simulink model "filecuaho"  (R2016b)
settings: Solver=VariableStepAuto  StartTime=0.0  StopTime=10.0  RelTol=1e-3
undefined symbols (not defined in the file): KACC_ACCT_CLR_NIDL_INIT, KACC_ACCUT_STATE_A, KACC_ACCUT_STATE_B, KACC_ACCUT_SW, KACC_ACTQSW, KACC_CLD, KACC_CLD_REQ_HYS, KACC_CLD_REQ_SW, KACC_COLPD, KACC_COMP_INRT, KACC_COMPTYPE_FIXED, KACC_COMPTYPE_VAR, KACC_CTTM_ACE, KACC_CTTM_ACON, KACC_CTTM_CRK, KACC_CTTM_FAN, KACC_CTTM_GRD, KACC_CTTM_IRS, KACC_CTTM_NAC, KACC_DIFFEVATEMPMAX, KACC_DIFFEVATEMPMIN, KACC_EVAT_ELSE, KACC_EVAT_ELSE_SW, KACC_EVATMPCUT_SW, KACC_EVATUPL_ELSE, KACC_EVATUPL_ELSE_SW, KACC_FANREQ_SW, KACC_FORCEDACON, KACC_HCAPS, KACC_HCAPS_HYS, KACC_HCCTTM, KACC_HCGRA, KACC_HCGRA_HYS, KACC_HCRGR, KACC_HCVS1, KACC_HCVS1_HYS, KACC_HCVS2, KACC_HCVS2_HYS, KACC_HEATUP_CE, KACC_HEATUP_CE_HYS, KACC_HEATUP_DRV2IDL, KACC_HEATUP_IDL2DRV, KACC_HEATUP_NE, KACC_HEATUP_NE_HYS, KACC_HIPS_ACOF, KACC_HIPS_ACON, KACC_LOPS_ACOF, KACC_LOPS_ACON, KACC_LYR3TR_ACHLD, KACC_NEW_RPM, KACC_OFDL_SW, KACC_OFDL_VCV, KACC_ONDL_SW, KACC_RECCP, KACC_RECCP_HYS, KACC_RECDLY, KACC_RECVS, KACC_S1_THWMAX, KACC_S1TM_THWULMT, KACC_SHLT_2CYL ... (+137)
libraries: lib2011b x727, SUBSYSTEM_LIB_CNV x30, SUBSYSTEM_LIB_ESC x2, SUBSYSTEM_LIB_AUX x1
(part 2 of 5)

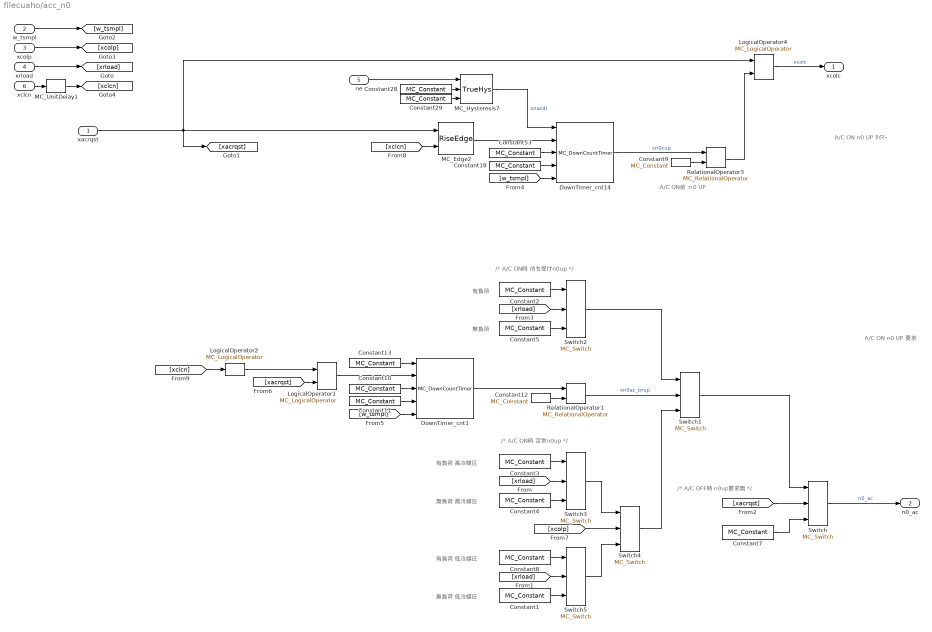
== system filecuaho/acc_n0 ==
  note: A/C ON前 ｎ0 UP
  note: A/C ON
      | n0 UP ﾀｲﾏｰ
  note: A/C ON
      | n0 UP 要求
  note: /* A/C ON時 待ち受けn0up */
  note: /* A/C ON時 定常n0up */
  note: /* A/C OFF時 n0up要求無 */
  note: 有負荷 高冷媒圧
  note: 無負荷 高冷媒圧
  note: 有負荷 低冷媒圧
  note: 無負荷 低冷媒圧
  note: 有負荷
  note: 無負荷
  xacrqst : Inport
  w_tsmpl : Inport  Port=2
  xcolp : Inport  Port=3
  xrload : Inport  Port=4
  ne : Inport  Port=5
  xclcn : Inport  Port=6
  Constant1 : lib2011b/Simulink Original/Sources/MC_Constant  Value=KINLCN  datatype=Inherit: Inherit from 'Constant value'  SampleTime=inf  FramePeriod=inf  OutMin=[]  OutMax=[]  OutDataTypeStr=Inherit: Inherit from 'Constant value'
  Constant10 : lib2011b/Simulink Original/Sources/MC_Constant  Value=true  datatype=Inherit: Inherit from 'Constant value'  SampleTime=inf  FramePeriod=inf  OutMin=[]  OutMax=[]  OutDataTypeStr=Inherit: Inherit from 'Constant value'
  Constant11 : lib2011b/Simulink Original/Sources/MC_Constant  Value=KLN0BRUP  datatype=Inherit: Inherit from 'Constant value'  SampleTime=inf  FramePeriod=inf  OutMin=[]  OutMax=[]  OutDataTypeStr=Inherit: Inherit from 'Constant value'
  Constant12 : lib2011b/Simulink Original/Sources/MC_Constant  Value=0  datatype=single  SampleTime=inf  FramePeriod=inf  OutMin=[]  OutMax=[]  OutDataTypeStr=single
  Constant13 : lib2011b/Simulink Original/Sources/MC_Constant  Value=false  datatype=Inherit: Inherit from 'Constant value'  SampleTime=inf  FramePeriod=inf  OutMin=[]  OutMax=[]  OutDataTypeStr=Inherit: Inherit from 'Constant value'
  Constant18 : lib2011b/Simulink Original/Sources/MC_Constant  Value=KLN0CUP  datatype=Inherit: Inherit from 'Constant value'  SampleTime=inf  FramePeriod=inf  OutMin=[]  OutMax=[]  OutDataTypeStr=Inherit: Inherit from 'Constant value'
  Constant2 : lib2011b/Simulink Original/Sources/MC_Constant  Value=KINLC1  datatype=Inherit: Inherit from 'Constant value'  SampleTime=inf  FramePeriod=inf  OutMin=[]  OutMax=[]  OutDataTypeStr=Inherit: Inherit from 'Constant value'
  Constant28 : lib2011b/Simulink Original/Sources/MC_Constant  Value=KSNACDL  datatype=Inherit: Inherit from 'Constant value'  SampleTime=inf  FramePeriod=inf  OutMin=[]  OutMax=[]  OutDataTypeStr=Inherit: Inherit from 'Constant value'
  Constant29 : lib2011b/Simulink Original/Sources/MC_Constant  Value=KSNACDL_HYS  datatype=Inherit: Inherit from 'Constant value'  SampleTime=inf  FramePeriod=inf  OutMin=[]  OutMax=[]  OutDataTypeStr=Inherit: Inherit from 'Constant value'
  Constant3 : lib2011b/Simulink Original/Sources/MC_Constant  Value=KINLCH  datatype=Inherit: Inherit from 'Constant value'  SampleTime=inf  FramePeriod=inf  OutMin=[]  OutMax=[]  OutDataTypeStr=Inherit: Inherit from 'Constant value'
  Constant4 : lib2011b/Simulink Original/Sources/MC_Constant  Value=KINLCHN  datatype=Inherit: Inherit from 'Constant value'  SampleTime=inf  FramePeriod=inf  OutMin=[]  OutMax=[]  OutDataTypeStr=Inherit: Inherit from 'Constant value'
  Constant5 : lib2011b/Simulink Original/Sources/MC_Constant  Value=KINLC1N  datatype=Inherit: Inherit from 'Constant value'  SampleTime=inf  FramePeriod=inf  OutMin=[]  OutMax=[]  OutDataTypeStr=Inherit: Inherit from 'Constant value'
  Constant53 : lib2011b/Simulink Original/Sources/MC_Constant  Value=true  datatype=Inherit: Inherit from 'Constant value'  SampleTime=inf  FramePeriod=inf  OutMin=[]  OutMax=[]  OutDataTypeStr=Inherit: Inherit from 'Constant value'
  Constant7 : lib2011b/Simulink Original/Sources/MC_Constant  Value=0  datatype=single  SampleTime=inf  FramePeriod=inf  OutMin=[]  OutMax=[]  OutDataTypeStr=single
  Constant8 : lib2011b/Simulink Original/Sources/MC_Constant  Value=KINLC  datatype=Inherit: Inherit from 'Constant value'  SampleTime=inf  FramePeriod=inf  OutMin=[]  OutMax=[]  OutDataTypeStr=Inherit: Inherit from 'Constant value'
  Constant9 : lib2011b/Simulink Original/Sources/MC_Constant  Value=0  datatype=single  SampleTime=inf  FramePeriod=inf  OutMin=[]  OutMax=[]  OutDataTypeStr=single
  DownTimer_cnt1 : lib2011b/Mazda Library/Timer/MC_DownCountTimer
      settings: AttributesFormatString=DownCountTimer
  DownTimer_cnt14 : lib2011b/Mazda Library/Timer/MC_DownCountTimer
      settings: AttributesFormatString=DownCountTimer
  LogicalOperator1 : lib2011b/Simulink Original/Logic and Bit Operations/MC_LogicalOperator  SelectedOperator=AND  Inputs=2  SampleTime=-1  AllPortsSameDT=off  OutDataTypeStr=boolean
  LogicalOperator2 : lib2011b/Simulink Original/Logic and Bit Operations/MC_LogicalOperator  SelectedOperator=NOT  Inputs=2  SampleTime=-1  AllPortsSameDT=off  OutDataTypeStr=boolean
  LogicalOperator4 : lib2011b/Simulink Original/Logic and Bit Operations/MC_LogicalOperator  SelectedOperator=AND  Inputs=2  SampleTime=-1  AllPortsSameDT=off  OutDataTypeStr=boolean
  MC_Edge2 : SUBSYSTEM_LIB_CNV/RiseEdge
      settings: AttributesFormatString=RISE
  MC_Hysteresis7 : SUBSYSTEM_LIB_CNV/TrueHys
      settings: AttributesFormatString=True
  MC_UnitDelay1 : lib2011b/Simulink Original/Discrete/MC_UnitDelay  InitialCondition=0  InputProcessing=Inherited  SampleTime=-1  StateName=delay_yclcn_b20m9489
      settings: StateMustResolveToSignalObject=off  StateStorageClass=ExportedGlobal
  RelationalOperator1 : lib2011b/Simulink Original/Logic and Bit Operations/MC_RelationalOperator  Operator=>  SampleTime=-1  InputSameDT=on  OutDataTypeStr=boolean
  RelationalOperator3 : lib2011b/Simulink Original/Logic and Bit Operations/MC_RelationalOperator  Operator=<=  SampleTime=-1  InputSameDT=on  OutDataTypeStr=boolean
  Switch{,1..5} (6 alike) : lib2011b/Simulink Original/Signal Routing/MC_Switch  Criteria=u2 ~= 0  Threshold=0  SampleTime=-1  InputSameDT=on  OutMin=[]  OutMax=[]  AllowDiffInputSizes=off
  xcolc : Outport
  n0_ac : Outport  Port=2
  wires:
  RelationalOperator3/1 -> LogicalOperator4/2
  Constant9/1 -> RelationalOperator3/2
  ne/1 -> MC_Hysteresis7/1
  Constant28/1 -> MC_Hysteresis7/2
  Constant29/1 -> MC_Hysteresis7/3
  xacrqst/1 -> MC_Edge2/1, LogicalOperator4/1, [xacrqst]
  MC_Edge2/1 -> DownTimer_cnt14/2
  MC_Hysteresis7/1 -> DownTimer_cnt14/1  "xnacdl"
  Constant18/1 -> DownTimer_cnt14/4
  Constant53/1 -> DownTimer_cnt14/3
  DownTimer_cnt14/1 -> RelationalOperator3/1  "cn0cup"
  Switch/1 -> n0_ac/1  "n0_ac"
  Switch5/1 -> Switch4/3
  Switch3/1 -> Switch4/1
  Constant8/1 -> Switch5/1
  Constant1/1 -> Switch5/3
  Constant7/1 -> Switch/3
  Constant3/1 -> Switch3/1
  Constant4/1 -> Switch3/3
  xrload/1 -> [xrload]
  [xrload] -> Switch3/2
  [xrload] -> Switch5/2
  [xacrqst] -> Switch/2
  Switch4/1 -> Switch1/3
  Switch1/1 -> Switch/1
  Constant2/1 -> Switch2/1
  [xrload] -> Switch2/2
  Constant5/1 -> Switch2/3
  w_tsmpl/1 -> [w_tsmpl]
  [w_tsmpl] -> DownTimer_cnt14/5
  [w_tsmpl] -> DownTimer_cnt1/5
  Constant10/1 -> DownTimer_cnt1/3
  Constant11/1 -> DownTimer_cnt1/4
  Constant12/1 -> RelationalOperator1/2
  DownTimer_cnt1/1 -> RelationalOperator1/1
  Constant13/1 -> DownTimer_cnt1/1
  LogicalOperator1/1 -> DownTimer_cnt1/2
  LogicalOperator2/1 -> LogicalOperator1/1
  [xacrqst] -> LogicalOperator1/2
  RelationalOperator1/1 -> Switch1/2  "xn0ac_brup"
  xcolp/1 -> [xcolp]
  [xcolp] -> Switch4/2
  Switch2/1 -> Switch1/1
  xclcn/1 -> MC_UnitDelay1/1
  [xclcn] -> LogicalOperator2/1
  MC_UnitDelay1/1 -> [xclcn]
  [xclcn] -> MC_Edge2/2
  LogicalOperator4/1 -> xcolc/1  "xcolc"

== system filecuaho/acc_nidle_enable ==
  note: << 暖房性能要求 N-Idle禁止制御 >>
  note: ②暖房性能要求熱量(リニアインテーク補正後)=0
  note: インマニ温(tham)センサ回路故障時は
      | インマニ温度履歴が正しくないため許可判定をキャンセルする
  note: ③センサ故障時
  note: ①インマニ温熱履歴条件
  note: 水温(thw)
      | ↑
      | ｜／／／／／／／／／／／／／／／／｜
      | ｜(B)エンジンルームの放熱量によらず
      | ｜N-IDLE許可可能領域／／／／／／／
      | ｜／／／／／／／／／／／／／／／／｜
      | ｜――――――――――――――――＋― TWNIDL_HEAT(_HYS)
      | ｜××××××××××××××××｜ 　　　↑
      | ｜(C)アイドル時のエンジンルームへの放熱量が　　暖房性能要求熱量=0
      | ｜少ない場合N-IDLE許可可能領域××　　　　(リニアインテーク補正後)
      | ｜××××××××××××××××｜　　 　↓
      | ｜――――――――――――――――＋――――――
      | ｜　　　　　　　　　　　　　　　　　　　　　　　　｜
      | ｜(D)暖房性能よりN-IDLE禁止領域　　　　　→(A)暖房性能からの要求無
      | ｜　　　　　　　　　　　　　　　　　　　　　　　　｜
      | ＋―――――――――――――――――――→始動時水温(thws)
      | 　　　　　　　　　　　　　　　　KWNIDL_HEAT_STA
  note: ----------------(B)エンジンルームの放熱量によらずN-IDLE許可可能領域----------------
  note: ----------------(C)アイドル時のエンジンルームへの放熱量が少ない場合N-IDLE許可可能領域----------------
  note: ----------------(A)暖房性能からのN-IDLE禁止要求無----------------
  note: 10000
  note: 1
  note: ②暖房性能要求熱量(リニアインテーク補正後)<=所定値
  thw : Inport
  thws : Inport  Port=2
  thaa : Inport  Port=3
  des_heat_acc_gain_drv : Inport  Port=4
  xheat_cldvvt_req : Inport  Port=5
  tham : Inport  Port=6
  xthamcf : Inport  Port=7
  vspe : Inport  Port=8
  xbrst : Inport  Port=9
  w_tsmpl : Inport  Port=10
  FalseHys : SUBSYSTEM_LIB_CNV/FalseHys
      settings: AttributesFormatString=False
  MC_Add : lib2011b/Simulink Original/Math Operations/MC_Add  Inputs=+-  CollapseDim=1  SampleTime=-1  InputSameDT=on  OutMin=[]  OutMax=[]  OutDataTypeStr=single
  MC_Constant1 : lib2011b/Simulink Original/Sources/MC_Constant  Value=KWNIDL_HEAT_GAIN_SW  datatype=Inherit: Inherit from 'Constant value'  SampleTime=inf  FramePeriod=inf  OutMin=[]  OutMax=[]  OutDataTypeStr=Inherit: Inherit from 'Constant value'
  MC_Constant14 : lib2011b/Simulink Original/Sources/MC_Constant  Value=KWNIDL_HEAT_GAIN2  datatype=Inherit: Inherit from 'Constant value'  SampleTime=inf  FramePeriod=inf  OutMin=[]  OutMax=[]  OutDataTypeStr=Inherit: Inherit from 'Constant value'
  MC_Constant16 : lib2011b/Simulink Original/Sources/MC_Constant  Value=KWNIDL_HEAT_GAIN2_HYS  datatype=Inherit: Inherit from 'Constant value'  SampleTime=inf  FramePeriod=inf  OutMin=[]  OutMax=[]  OutDataTypeStr=Inherit: Inherit from 'Constant value'
  MC_Constant2 : lib2011b/Simulink Original/Sources/MC_Constant  Value=KWNIDL_HEAT_STA  datatype=Inherit: Inherit from 'Constant value'  SampleTime=inf  FramePeriod=inf  OutMin=[]  OutMax=[]  OutDataTypeStr=Inherit: Inherit from 'Constant value'
  MC_Constant3 : lib2011b/Simulink Original/Sources/MC_Constant  Value=KWNIDL_HEAT_GAIN  datatype=Inherit: Inherit from 'Constant value'  SampleTime=inf  FramePeriod=inf  OutMin=[]  OutMax=[]  OutDataTypeStr=Inherit: Inherit from 'Constant value'
  MC_Constant4 : lib2011b/Simulink Original/Sources/MC_Constant  Value=KWNIDL_HEAT_HYS  datatype=Inherit: Inherit from 'Constant value'  SampleTime=inf  FramePeriod=inf  OutMin=[]  OutMax=[]  OutDataTypeStr=Inherit: Inherit from 'Constant value'
  MC_Constant6 : lib2011b/Simulink Original/Sources/MC_Constant  Value=KWNIDL_LATCH_VSP  datatype=Inherit: Inherit from 'Constant value'  SampleTime=inf  FramePeriod=inf  OutMin=[]  OutMax=[]  OutDataTypeStr=Inherit: Inherit from 'Constant value'
  MC_Constant7 : lib2011b/Simulink Original/Sources/MC_Constant  Value=KWNIDL_THAM_FIL_TC  datatype=Inherit: Inherit from 'Constant value'  SampleTime=inf  FramePeriod=inf  OutMin=[]  OutMax=[]  OutDataTypeStr=Inherit: Inherit from 'Constant value'
  MC_DataTypeConversion1 : lib2011b/Simulink Original/Signal Attributes/MC_DataTypeConversion  OutMin=[]  OutMax=[]  OutDataTypeStr=boolean  Signaltype=boolean  ConvertRealWorld=Real World Value (RWV)  RndMeth=Zero  SaturateOnIntegerOverflow=on  SampleTime=-1
  MC_Hysteresis : SUBSYSTEM_LIB_CNV/TrueHys
      settings: AttributesFormatString=True
  MC_LogicalOperator1 : lib2011b/Simulink Original/Logic and Bit Operations/MC_LogicalOperator  SelectedOperator=AND  Inputs=3  SampleTime=-1  AllPortsSameDT=off  OutDataTypeStr=boolean
  MC_LogicalOperator2 : lib2011b/Simulink Original/Logic and Bit Operations/MC_LogicalOperator  SelectedOperator=NOT  Inputs=1  SampleTime=-1  AllPortsSameDT=off  OutDataTypeStr=boolean
  MC_LogicalOperator3 : lib2011b/Simulink Original/Logic and Bit Operations/MC_LogicalOperator  SelectedOperator=OR  Inputs=3  SampleTime=-1  AllPortsSameDT=off  OutDataTypeStr=boolean
  MC_LogicalOperator4 : lib2011b/Simulink Original/Logic and Bit Operations/MC_LogicalOperator  SelectedOperator=OR  Inputs=2  SampleTime=-1  AllPortsSameDT=off  OutDataTypeStr=boolean
  MC_LogicalOperator6 : lib2011b/Simulink Original/Logic and Bit Operations/MC_LogicalOperator  SelectedOperator=NOT  Inputs=1  SampleTime=-1  AllPortsSameDT=off  OutDataTypeStr=boolean
  MC_LowPassFilter : lib2011b/Mazda Library/Filter/MC_LowPassFilter
  MC_MinMax : lib2011b/Simulink Original/Math Operations/MC_MinMax  Function=min  Inputs=2  SampleTime=-1  InputSameDT=on  OutMin=[]  OutMax=[]
  MC_MinMax1 : lib2011b/Simulink Original/Math Operations/MC_MinMax  Function=min  Inputs=2  SampleTime=-1  InputSameDT=on  OutMin=[]  OutMax=[]
  MC_RelationalOperator : lib2011b/Simulink Original/Logic and Bit Operations/MC_RelationalOperator  Operator=>=  SampleTime=-1  InputSameDT=on  OutDataTypeStr=boolean
  MC_RelationalOperator1 : lib2011b/Simulink Original/Logic and Bit Operations/MC_RelationalOperator  Operator=<=  SampleTime=-1  InputSameDT=on  OutDataTypeStr=boolean
  MC_RelationalOperator2 : lib2011b/Simulink Original/Logic and Bit Operations/MC_RelationalOperator  Operator=>=  SampleTime=-1  InputSameDT=on  OutDataTypeStr=boolean
  MC_RelationalOperator4 : lib2011b/Simulink Original/Logic and Bit Operations/MC_RelationalOperator  Operator=>=  SampleTime=-1  InputSameDT=on  OutDataTypeStr=boolean
  MC_Switch1 : lib2011b/Simulink Original/Signal Routing/MC_Switch  Criteria=u2 ~= 0  Threshold=0  SampleTime=-1  InputSameDT=on  OutMin=[]  OutMax=[]  AllowDiffInputSizes=off
  MC_Switch2 : lib2011b/Simulink Original/Signal Routing/MC_Switch  Criteria=u2 ~= 0  Threshold=0  SampleTime=-1  InputSameDT=on  OutMin=[]  OutMax=[]  AllowDiffInputSizes=off
  MC_Table : lib2011b/Simulink Original/Lookup Tables/MC_Table_i  Label=TWNIDL_HEAT  InputValues=TWNIDL_HEAT_X  calsw_x=on  OutputValues=TWNIDL_HEAT_Y  LsbValue=LSB_TWNIDL_HEAT_Y  OffsetValue=OFFSET_TWNIDL_HEAT_Y
      settings: AttributesFormatString=%<Label>\nX-axis %<calsw_x>
  MC_Table1 : lib2011b/Simulink Original/Lookup Tables/MC_Table_i  Label=TWNIDL_DLT_THAM  InputValues=TWNIDL_DLT_THAM_X  calsw_x=on  OutputValues=TWNIDL_DLT_THAM_Y  LsbValue=LSB_TWNIDL_DLT_THAM_Y  OffsetValue=OFFSET_TWNIDL_DLT_THAM_Y
      settings: AttributesFormatString=%<Label>\nX-axis %<calsw_x>
  MC_UnitDelay : lib2011b/Simulink Original/Discrete/MC_UnitDelay  InitialCondition=0  InputProcessing=Inherited  SampleTime=-1  StateName=delay_yclcn_b20m9490
      settings: StateMustResolveToSignalObject=off  StateStorageClass=ExportedGlobal
  MC_UnitDelay1 : lib2011b/Simulink Original/Discrete/MC_UnitDelay  InitialCondition=0  InputProcessing=Inherited  SampleTime=-1  StateName=delay_yclcn_b20m9491
      settings: StateMustResolveToSignalObject=off  StateStorageClass=ExportedGlobal
  MC_UnitDelay3 : lib2011b/Simulink Original/Discrete/MC_UnitDelay  InitialCondition=0  InputProcessing=Inherited  SampleTime=-1  StateName=delay_yclcn_b20m9492
      settings: StateMustResolveToSignalObject=off  StateStorageClass=ExportedGlobal
  xnidle_ena_heat : Outport
  wires:
  thw/1 -> [thw]
  MC_Table/1 -> MC_Hysteresis/2
  MC_Constant4/1 -> MC_Hysteresis/3
  MC_Hysteresis/1 -> MC_LogicalOperator3/2
  thws/1 -> [thws]
  MC_Constant2/1 -> MC_RelationalOperator/2
  MC_RelationalOperator/1 -> MC_LogicalOperator3/1
  MC_MinMax/1 -> MC_Table/1, MC_UnitDelay/1
  thaa/1 -> MC_MinMax/1
  MC_UnitDelay/1 -> MC_MinMax/2
  MC_LogicalOperator3/1 -> xnidle_ena_heat/1  "xnidle_ena_heat"
  MC_UnitDelay1/1 -> MC_MinMax1/2
  MC_LowPassFilter/1 -> MC_MinMax1/1, MC_Add/1  "tham_fil_heat"
  MC_MinMax1/1 -> MC_UnitDelay1/1, MC_Add/2
  [thw] -> MC_Hysteresis/1
  [thws] -> MC_RelationalOperator/1
  MC_Add/1 -> MC_RelationalOperator2/1
  xthamcf/1 -> MC_LogicalOperator6/1
  MC_LogicalOperator6/1 -> MC_LogicalOperator1/3
  MC_Constant7/1 -> MC_LowPassFilter/2
  xbrst/1 -> MC_LowPassFilter/4
  w_tsmpl/1 -> MC_LowPassFilter/3
  tham/1 -> MC_LowPassFilter/1
  MC_Switch2/1 -> MC_UnitDelay3/1, MC_LogicalOperator3/3
  MC_UnitDelay3/1 -> MC_Switch2/3
  vspe/1 -> MC_RelationalOperator4/1
  MC_RelationalOperator4/1 -> MC_Switch2/2
  MC_Constant6/1 -> MC_RelationalOperator4/2
  xheat_cldvvt_req/1 -> MC_LogicalOperator2/1
  MC_Table1/1 -> MC_RelationalOperator2/2
  MC_RelationalOperator2/1 -> MC_LogicalOperator1/1
  MC_LogicalOperator1/1 -> MC_Switch2/1
  [thws] -> MC_Table1/1
  MC_Constant1/1 -> MC_DataTypeConversion1/1
  MC_DataTypeConversion1/1 -> MC_Switch1/2
  MC_Constant14/1 -> FalseHys/2
  MC_Constant16/1 -> FalseHys/3
  des_heat_acc_gain_drv/1 -> FalseHys/1, MC_RelationalOperator1/1
  MC_LogicalOperator4/1 -> MC_Switch1/1
  FalseHys/1 -> MC_LogicalOperator4/1
  MC_RelationalOperator1/1 -> MC_LogicalOperator4/2
  MC_Constant3/1 -> MC_RelationalOperator1/2
  MC_LogicalOperator2/1 -> MC_Switch1/3
  MC_Switch1/1 -> MC_LogicalOperator1/2

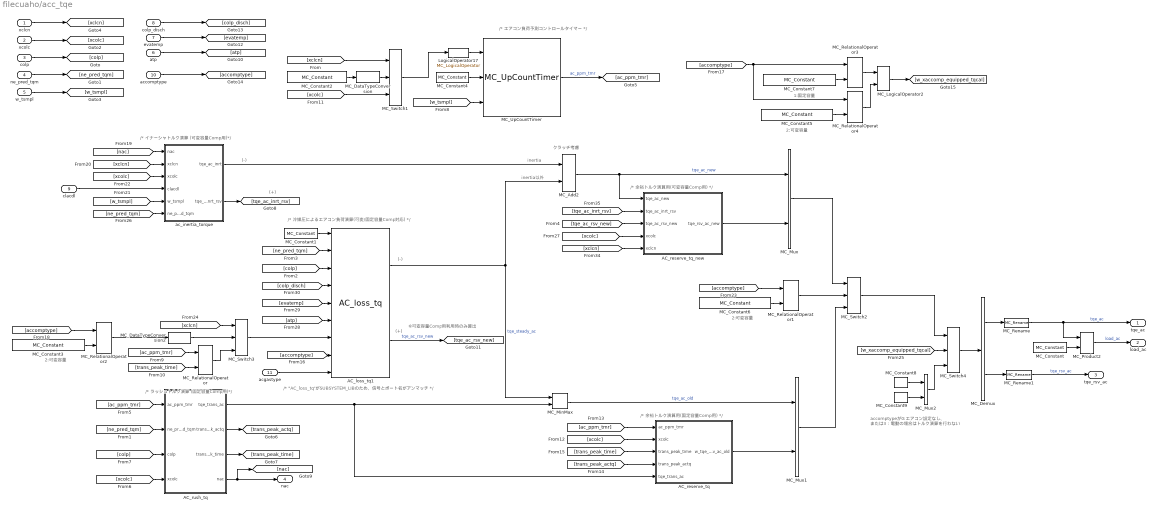
== system filecuaho/acc_tqe ==
  note: /* エアコン負荷予測コントロールタイマー */
  note: /* ラッシュトルク演算 (固定容量Comp用)*/
  note: /* 冷媒圧によるエアコン負荷演算(可変/固定容量Comp対応) */
  note: /* "AC_loss_tq"がSUBSYSTEM_LIBのため、信号とポート名がアンマッチ */
  note: /* 余裕トルク演算用(固定容量Comp用) */
  note: クラッチ考慮
  note: /* イナーシャトルク演算 (可変容量Comp用)*/
  note: inertia
  note: inertia以外
  note: (+)
  note: (-)
  note: (+)
  note: (-)
  note: /* 余裕トルク演算用(可変容量Comp用) */
  note: ※可変容量Comp用利用時のみ算出
  note: 2:可変容量
  note: 2:可変容量
  note: 2:可変容量
  note: 1:固定容量
  note: accomptypeが0:エアコン設定なし、
      | または3：電動の場合はトルク演算を行わない
  xclcn : Inport
  xcolc : Inport  Port=2
  colp : Inport  Port=3
  ne_pred_tqm : Inport  Port=4
  w_tsmpl : Inport  Port=5
  atp : Inport  Port=6
  evatemp : Inport  Port=7
  colp_disch : Inport  Port=8
  clacdl : Inport  Port=9
  accomptype : Inport  Port=10
  acgastype : Inport  Port=11
  AC_loss_tq1 : SUBSYSTEM_LIB_AUX/ACC/AC_loss_tq
  AC_reserve_tq : Subsystem
  AC_reserve_tq_new : Subsystem
  AC_rush_tq : Subsystem
  LogicalOperator17 : lib2011b/Simulink Original/Logic and Bit Operations/MC_LogicalOperator  SelectedOperator=NOT  Inputs=1  SampleTime=-1  AllPortsSameDT=off  OutDataTypeStr=boolean
  MC_Add2 : lib2011b/Simulink Original/Math Operations/MC_Add  Inputs=++  CollapseDim=1  SampleTime=-1  InputSameDT=on  OutMin=[]  OutMax=[]  OutDataTypeStr=single
  MC_Constant : lib2011b/Simulink Original/Sources/MC_Constant  Value=-1  datatype=single  SampleTime=inf  FramePeriod=inf  OutMin=[]  OutMax=[]  OutDataTypeStr=single
  MC_Constant1 : lib2011b/Simulink Original/Sources/MC_Constant  Value=1  datatype=single  SampleTime=inf  FramePeriod=inf  OutMin=[]  OutMax=[]  OutDataTypeStr=single
  MC_Constant2 : lib2011b/Simulink Original/Sources/MC_Constant  Value=KACC_ACTQSW  datatype=Inherit: Inherit from 'Constant value'  SampleTime=inf  FramePeriod=inf  OutMin=[]  OutMax=[]  OutDataTypeStr=Inherit: Inherit from 'Constant value'
  MC_Constant3 : lib2011b/Simulink Original/Sources/MC_Constant  Value=KACC_COMPTYPE_VAR  datatype=Inherit: Inherit from 'Constant value'  SampleTime=inf  FramePeriod=inf  OutMin=[]  OutMax=[]  OutDataTypeStr=Inherit: Inherit from 'Constant value'
  MC_Constant4 : lib2011b/Simulink Original/Sources/MC_Constant  Value=true  datatype=Inherit: Inherit from 'Constant value'  SampleTime=inf  FramePeriod=inf  OutMin=[]  OutMax=[]  OutDataTypeStr=Inherit: Inherit from 'Constant value'
  MC_Constant5 : lib2011b/Simulink Original/Sources/MC_Constant  Value=KACC_COMPTYPE_VAR  datatype=Inherit: Inherit from 'Constant value'  SampleTime=inf  FramePeriod=inf  OutMin=[]  OutMax=[]  OutDataTypeStr=Inherit: Inherit from 'Constant value'
  MC_Constant6 : lib2011b/Simulink Original/Sources/MC_Constant  Value=KACC_COMPTYPE_VAR  datatype=Inherit: Inherit from 'Constant value'  SampleTime=inf  FramePeriod=inf  OutMin=[]  OutMax=[]  OutDataTypeStr=Inherit: Inherit from 'Constant value'
  MC_Constant7 : lib2011b/Simulink Original/Sources/MC_Constant  Value=KACC_COMPTYPE_FIXED  datatype=Inherit: Inherit from 'Constant value'  SampleTime=inf  FramePeriod=inf  OutMin=[]  OutMax=[]  OutDataTypeStr=Inherit: Inherit from 'Constant value'
  MC_Constant8 : lib2011b/Simulink Original/Sources/MC_Constant  Value=0  datatype=single  SampleTime=inf  FramePeriod=inf  OutMin=[]  OutMax=[]  OutDataTypeStr=single
  MC_Constant9 : lib2011b/Simulink Original/Sources/MC_Constant  Value=0  datatype=single  SampleTime=inf  FramePeriod=inf  OutMin=[]  OutMax=[]  OutDataTypeStr=single
  MC_DataTypeConversion : lib2011b/Simulink Original/Signal Attributes/MC_DataTypeConversion  OutMin=[]  OutMax=[]  OutDataTypeStr=boolean  Signaltype=boolean  ConvertRealWorld=Real World Value (RWV)  RndMeth=Zero  SampleTime=-1
  MC_DataTypeConversion2 : lib2011b/Simulink Original/Signal Attributes/MC_DataTypeConversion  OutMin=[]  OutMax=[]  OutDataTypeStr=boolean  Signaltype=boolean  ConvertRealWorld=Real World Value (RWV)  RndMeth=Zero  SampleTime=-1
  MC_Demux : lib2011b/Simulink Original/Signal Routing/MC_Demux  Outputs=2  BusSelectionMode=off
  MC_LogicalOperator2 : lib2011b/Simulink Original/Logic and Bit Operations/MC_LogicalOperator  SelectedOperator=OR  Inputs=2  SampleTime=-1  AllPortsSameDT=off  OutDataTypeStr=boolean
  MC_MinMax : lib2011b/Simulink Original/Math Operations/MC_MinMax  Function=min  Inputs=2  SampleTime=-1  InputSameDT=on  OutMin=[]  OutMax=[]
  MC_Mux : lib2011b/Simulink Original/Signal Routing/MC_Mux  Inputs=2
  MC_Mux1 : lib2011b/Simulink Original/Signal Routing/MC_Mux  Inputs=2
  MC_Mux2 : lib2011b/Simulink Original/Signal Routing/MC_Mux  Inputs=2
  MC_Product2 : lib2011b/Simulink Original/Math Operations/MC_Product  Inputs=**  Multiplication=Element-wise(.*)  CollapseDim=1  SampleTime=-1  OutMin=[]  OutMax=[]  OutDataTypeStr=single  RndMeth=Zero
  MC_RelationalOperator : lib2011b/Simulink Original/Logic and Bit Operations/MC_RelationalOperator  Operator=>  SampleTime=-1  InputSameDT=on  OutDataTypeStr=boolean
  MC_RelationalOperator{1..4} (4 alike) : lib2011b/Simulink Original/Logic and Bit Operations/MC_RelationalOperator  Operator===  SampleTime=-1  InputSameDT=on  OutDataTypeStr=boolean
  MC_Rename : lib2011b/Mazda Library/Other/MC_Rename
  MC_Rename1 : lib2011b/Mazda Library/Other/MC_Rename
  MC_Switch{1..4} (4 alike) : lib2011b/Simulink Original/Signal Routing/MC_Switch  Criteria=u2 ~= 0  Threshold=0  SampleTime=-1  InputSameDT=on  OutMin=[]  OutMax=[]  AllowDiffInputSizes=off
  MC_UpCountTimer : lib2011b/Mazda Library/Timer/MC_UpCountTimer  tmax=2147483647  tmax_bg=2147483647
      settings: AttributesFormatString=UpCountTimer\nMAX = %<tmax>ms
  ac_inertia_torque : Subsystem
  tqe_ac : Outport
  load_ac : Outport  Port=2
  tqe_rsv_ac : Outport  Port=3
  nac : Outport  Port=4
  wires:
  MC_Product2/1 -> load_ac/1  "load_ac"
  MC_Constant/1 -> MC_Product2/2
  LogicalOperator17/1 -> MC_UpCountTimer/1
  colp/1 -> [colp]
  ne_pred_tqm/1 -> [ne_pred_tqm]
  [ne_pred_tqm] -> AC_rush_tq/2(ne_pred_tqm)
  [colp] -> AC_loss_tq1/3
  [ne_pred_tqm] -> AC_loss_tq1/2
  xcolc/1 -> [xcolc]
  [colp] -> AC_rush_tq/3(colp)
  [xcolc] -> AC_rush_tq/4(xcolc)
  w_tsmpl/1 -> [w_tsmpl]
  [w_tsmpl] -> MC_UpCountTimer/3
  xclcn/1 -> [xclcn]
  MC_UpCountTimer/1 -> [ac_ppm_tmr]  "ac_ppm_tmr"
  MC_Constant1/1 -> AC_loss_tq1/1
  AC_rush_tq/1(tqe_trans_ac) -> AC_reserve_tq/5(tqe_trans_ac), MC_MinMax/2
  AC_loss_tq1/1 -> MC_MinMax/1, MC_Add2/2  "tqe_steady_ac"
  MC_Rename/1 -> tqe_ac/1, MC_Product2/1  "tqe_ac"
  [ac_ppm_tmr] -> AC_rush_tq/1(ac_ppm_tmr)
  [ac_ppm_tmr] -> MC_RelationalOperator/1
  AC_rush_tq/2(trans_peak_actq) -> [trans_peak_actq]
  AC_rush_tq/3(trans_peak_time) -> [trans_peak_time]
  [trans_peak_time] -> MC_RelationalOperator/2
  AC_reserve_tq/1(w_tqe_rsv_ac_old) -> MC_Mux1/2
  [ac_ppm_tmr] -> AC_reserve_tq/1(ac_ppm_tmr)
  [xcolc] -> AC_reserve_tq/2(xcolc)
  [trans_peak_time] -> AC_reserve_tq/3(trans_peak_time)
  MC_Switch1/1 -> LogicalOperator17/1
  [xclcn] -> MC_Switch1/1
  [xcolc] -> MC_Switch1/3
  MC_Constant2/1 -> MC_DataTypeConversion/1
  MC_DataTypeConversion/1 -> MC_Switch1/2
  AC_rush_tq/4(nac) -> nac/1, [nac]
  [nac] -> ac_inertia_torque/1(nac)
  [xclcn] -> ac_inertia_torque/2(xclcn)
  MC_MinMax/1 -> MC_Mux1/1  "tqe_ac_old"
  MC_RelationalOperator1/1 -> MC_Switch2/2
  [w_tsmpl] -> ac_inertia_torque/5(w_tsmpl)
  [xcolc] -> ac_inertia_torque/3(xcolc)
  clacdl/1 -> ac_inertia_torque/4(clacdl)
  MC_Constant4/1 -> MC_UpCountTimer/2
  MC_DataTypeConversion2/1 -> MC_Switch3/2
  [xclcn] -> MC_Switch3/1
  MC_RelationalOperator/1 -> MC_Switch3/3
  [colp_disch] -> AC_loss_tq1/4
  [evatemp] -> AC_loss_tq1/5
  [atp] -> AC_loss_tq1/6
  MC_Switch3/1 -> AC_loss_tq1/7
  ac_inertia_torque/1(tqe_ac_inrt) -> MC_Add2/1
  MC_Add2/1 -> MC_Mux/1, AC_reserve_tq_new/1(tqe_ac_new)  "tqe_ac_new"
  AC_loss_tq1/2 -> [tqe_ac_rsv_new]  "tqe_ac_rsv_new"
  ac_inertia_torque/2(tqe_ac_inrt_rsv) -> [tqe_ac_inrt_rsv]
  MC_Rename1/1 -> tqe_rsv_ac/1  "tqe_rsv_ac"
  [xcolc] -> AC_reserve_tq_new/4(xcolc)
  [tqe_ac_inrt_rsv] -> AC_reserve_tq_new/2(tqe_ac_inrt_rsv)
  [tqe_ac_rsv_new] -> AC_reserve_tq_new/3(tqe_ac_rsv_new)
  [xclcn] -> AC_reserve_tq_new/5(xclcn)
  AC_reserve_tq_new/1(tqe_rsv_ac_new) -> MC_Mux/2
  MC_Mux/1 -> MC_Switch2/1
  [trans_peak_actq] -> AC_reserve_tq/4(trans_peak_actq)
  MC_Mux1/1 -> MC_Switch2/3
  colp_disch/1 -> [colp_disch]
  evatemp/1 -> [evatemp]
  atp/1 -> [atp]
  MC_Demux/1 -> MC_Rename/1
  MC_Demux/2 -> MC_Rename1/1
  [accomptype] -> AC_loss_tq1/8
  acgastype/1 -> AC_loss_tq1/9
  MC_Constant6/1 -> MC_RelationalOperator1/2
  accomptype/1 -> [accomptype]
  [accomptype] -> MC_RelationalOperator1/1
  MC_RelationalOperator2/1 -> MC_DataTypeConversion2/1
  MC_Constant3/1 -> MC_RelationalOperator2/2
  [accomptype] -> MC_RelationalOperator2/1
  MC_RelationalOperator4/1 -> MC_LogicalOperator2/2
  MC_RelationalOperator3/1 -> MC_LogicalOperator2/1
  MC_Constant5/1 -> MC_RelationalOperator4/2
  MC_Constant7/1 -> MC_RelationalOperator3/2
  [accomptype] -> MC_RelationalOperator3/1, MC_RelationalOperator4/1
  MC_Constant8/1 -> MC_Mux2/1
  MC_Constant9/1 -> MC_Mux2/2
  MC_LogicalOperator2/1 -> [w_xaccomp_equipped_tqcal]
  MC_Switch4/1 -> MC_Demux/1
  MC_Switch2/1 -> MC_Switch4/1
  [w_xaccomp_equipped_tqcal] -> MC_Switch4/2
  MC_Mux2/1 -> MC_Switch4/3
  [ne_pred_tqm] -> ac_inertia_torque/6(ne_pred_tqm)

== system filecuaho/acc_xaccuton ==
  w_tsmpl : Inport
  xbrst : Inport  Port=2
  xzst : Inport  Port=3
  ne : Inport  Port=4
  gearp : Inport  Port=5
  apsfil : Inport  Port=6
  xrload : Inport  Port=7
  xaltcalflg : Inport  Port=8
  colp : Inport  Port=9
  xfsacih : Inport  Port=10
  w_xsdpan : Inport  Port=11
  xidld : Inport  Port=12
  xcol : Inport  Port=13
  xhpr_accut : Inport  Port=14
  xclcn : Inport  Port=15
  vspe : Inport  Port=16
  xstbymd_iss : Inport  Port=17
  xismd_iss : Inport  Port=18
  xirmd_iss : Inport  Port=19
  rgear : Inport  Port=20
  grade : Inport  Port=21
  xvspf : Inport  Port=22
  evatemp_uplmt : Inport  Port=23
  evatemp : Inport  Port=24
  iss_state : Inport  Port=25
  xclcncf : Inport  Port=26
  xacptc2f : Inport  Port=27
  vcv_cut_time : Inport  Port=28
  xnlidl : Inport  Port=29
  acc_accutreq : Subsystem
      mask Display: disp('A/Cカット要求')
  xaccuton : Outport
  xemg_hldclr : Outport  Port=2
  xacct1 : Outport  Port=3
  xcolp : Outport  Port=4
  xlacfs : Outport  Port=5
  xemg_accut : Outport  Port=6
  wires:
  w_tsmpl/1 -> acc_accutreq/1(w_tsmpl)
  xbrst/1 -> acc_accutreq/2(xbrst)
  xzst/1 -> acc_accutreq/3(xzst)
  ne/1 -> acc_accutreq/4(ne)
  gearp/1 -> acc_accutreq/5(gearp)
  apsfil/1 -> acc_accutreq/6(apsfil)
  xrload/1 -> acc_accutreq/7(xrload)
  xaltcalflg/1 -> acc_accutreq/8(xaltcalflg)
  colp/1 -> acc_accutreq/9(colp)
  xfsacih/1 -> acc_accutreq/10(xfsacih)
  w_xsdpan/1 -> acc_accutreq/11(w_xsdpan)
  xidld/1 -> acc_accutreq/12(xidld)
  xcol/1 -> acc_accutreq/13(xcol)
  xhpr_accut/1 -> acc_accutreq/14(xhpr_accut)
  xclcn/1 -> acc_accutreq/15(xclcn)
  vspe/1 -> acc_accutreq/16(vspe)
  xstbymd_iss/1 -> acc_accutreq/17(xstbymd_iss)
  xismd_iss/1 -> acc_accutreq/18(xismd_iss)
  xirmd_iss/1 -> acc_accutreq/19(xirmd_iss)
  acc_accutreq/1(xaccuton) -> xaccuton/1
  acc_accutreq/2(xacct1) -> xacct1/1
  acc_accutreq/3(xcolp) -> xcolp/1
  rgear/1 -> acc_accutreq/20(rgear)
  grade/1 -> acc_accutreq/21(grade)
  xvspf/1 -> acc_accutreq/22(xvspf)
  acc_accutreq/4(xemg_hldclr) -> xemg_hldclr/1
  acc_accutreq/5(xlacfs) -> xlacfs/1
  evatemp_uplmt/1 -> acc_accutreq/23(evatemp_uplmt)
  evatemp/1 -> acc_accutreq/24(evatemp)
  iss_state/1 -> acc_accutreq/25(iss_state)
  xclcncf/1 -> acc_accutreq/26(xclcncf)
  acc_accutreq/6(xemg_accut) -> xemg_accut/1
  xacptc2f/1 -> acc_accutreq/27(xacptc2f)
  vcv_cut_time/1 -> acc_accutreq/28(vcv_cut_time)
  xnlidl/1 -> acc_accutreq/29(xnlidl)

== system filecuaho/acc_xacrec ==
  colp : Inport
  vspe : Inport  Port=2
  xidld : Inport  Port=3
  w_tsmpl : Inport  Port=4
  MC_Constant : lib2011b/Simulink Original/Sources/MC_Constant  Value=KACC_RECCP  datatype=Inherit: Inherit from 'Constant value'  SampleTime=inf  FramePeriod=inf  OutMin=[]  OutMax=[]  OutDataTypeStr=Inherit: Inherit from 'Constant value'
  MC_Constant1 : lib2011b/Simulink Original/Sources/MC_Constant  Value=KACC_RECCP_HYS  datatype=Inherit: Inherit from 'Constant value'  SampleTime=inf  FramePeriod=inf  OutMin=[]  OutMax=[]  OutDataTypeStr=Inherit: Inherit from 'Constant value'
  MC_Constant2 : lib2011b/Simulink Original/Sources/MC_Constant  Value=KACC_RECVS  datatype=Inherit: Inherit from 'Constant value'  SampleTime=inf  FramePeriod=inf  OutMin=[]  OutMax=[]  OutDataTypeStr=Inherit: Inherit from 'Constant value'
  MC_Constant3 : lib2011b/Simulink Original/Sources/MC_Constant  Value=KACC_RECDLY  datatype=Inherit: Inherit from 'Constant value'  SampleTime=inf  FramePeriod=inf  OutMin=[]  OutMax=[]  OutDataTypeStr=Inherit: Inherit from 'Constant value'
  MC_Constant4 : lib2011b/Simulink Original/Sources/MC_Constant  Value=0  datatype=single  SampleTime=inf  FramePeriod=inf  OutMin=[]  OutMax=[]  OutDataTypeStr=single
  MC_DownCounter : lib2011b/Mazda Library/Counter/MC_DownCounter  EnblRst=off
      settings: AttributesFormatString=Down Counter
  MC_Hysteresis : SUBSYSTEM_LIB_CNV/TrueHys
      settings: AttributesFormatString=True
  MC_LogicalOperator : lib2011b/Simulink Original/Logic and Bit Operations/MC_LogicalOperator  SelectedOperator=AND  Inputs=2  SampleTime=-1  AllPortsSameDT=off  OutDataTypeStr=boolean
  MC_LogicalOperator1 : lib2011b/Simulink Original/Logic and Bit Operations/MC_LogicalOperator  SelectedOperator=NOT  Inputs=2  SampleTime=-1  AllPortsSameDT=off  OutDataTypeStr=boolean
  MC_LogicalOperator2 : lib2011b/Simulink Original/Logic and Bit Operations/MC_LogicalOperator  SelectedOperator=AND  Inputs=2  SampleTime=-1  AllPortsSameDT=off  OutDataTypeStr=boolean
  MC_Product : lib2011b/Simulink Original/Math Operations/MC_Product  Inputs=*/  Multiplication=Element-wise(.*)  CollapseDim=1  SampleTime=-1  OutMin=[]  OutMax=[]  OutDataTypeStr=single  RndMeth=Zero
  MC_RelationalOperator : lib2011b/Simulink Original/Logic and Bit Operations/MC_RelationalOperator  Operator=<=  SampleTime=-1  InputSameDT=on  OutDataTypeStr=boolean
  MC_RelationalOperator1 : lib2011b/Simulink Original/Logic and Bit Operations/MC_RelationalOperator  Operator=>  SampleTime=-1  InputSameDT=on  OutDataTypeStr=boolean
  xacrec : Outport
  wires:
  colp/1 -> MC_Hysteresis/1
  MC_Constant/1 -> MC_Hysteresis/2
  MC_Constant1/1 -> MC_Hysteresis/3
  vspe/1 -> MC_RelationalOperator/1
  MC_Constant2/1 -> MC_RelationalOperator/2
  MC_RelationalOperator/1 -> MC_LogicalOperator/1
  xidld/1 -> MC_LogicalOperator/2
  MC_LogicalOperator/1 -> MC_DownCounter/1, MC_LogicalOperator1/1
  MC_LogicalOperator1/1 -> MC_DownCounter/2
  MC_Product/1 -> MC_DownCounter/3
  MC_Constant3/1 -> MC_Product/1
  w_tsmpl/1 -> MC_Product/2
  MC_Hysteresis/1 -> MC_LogicalOperator2/1  "xcolacrec"
  MC_LogicalOperator2/1 -> xacrec/1  "xacrec"
  MC_DownCounter/1 -> MC_RelationalOperator1/1  "cacrecvdly"
  MC_Constant4/1 -> MC_RelationalOperator1/2
  MC_RelationalOperator1/1 -> MC_LogicalOperator2/2

== system filecuaho/acc_xcol ==
  note: A/C SW入力（CAN）
  xcolcan : Inport
  MC_Rename : lib2011b/Mazda Library/Other/MC_Rename
  MC_Rename1 : lib2011b/Mazda Library/Other/MC_Rename
  xcol : Outport
  xdid_099b_b08_r : Outport  Port=2
  wires:
  MC_Rename1/1 -> xcol/1  "xcol"
  MC_Rename/1 -> xdid_099b_b08_r/1  "xdid_099b_b08_r"
  xcolcan/1 -> MC_Rename1/1, MC_Rename/1

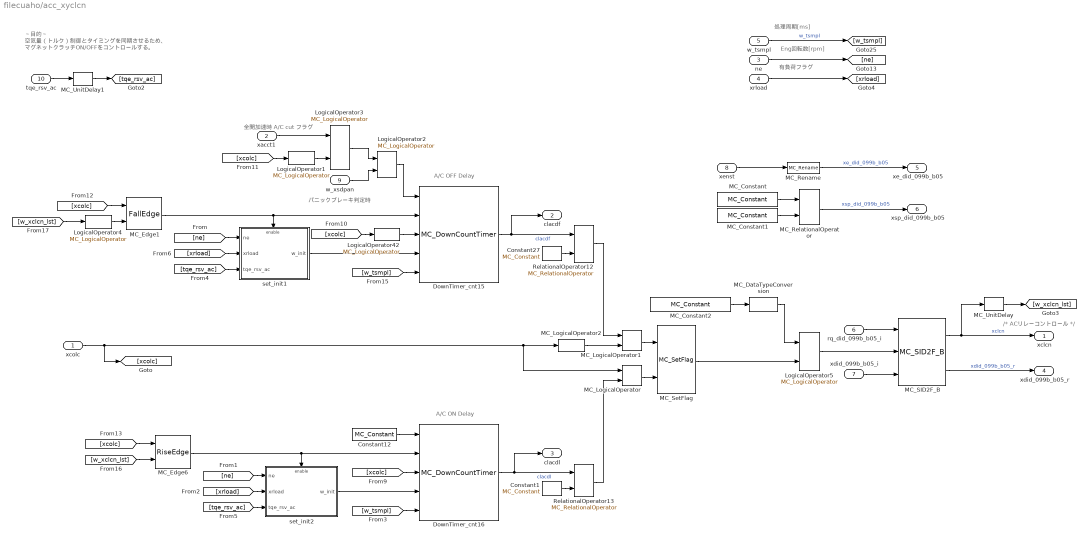
== system filecuaho/acc_xyclcn ==
  note: パニックブレーキ判定時
  note: 処理周期[ms]
  note: Eng回転数[rpm]
  note: 有負荷フラグ
  note: 全開加速時
      | A/C cut フラグ
  note: /* ACリレーコントロール */
  note: A/C ON Delay
  note: A/C OFF Delay
  note: ～目的～
      | 空気量（トルク）制御とタイミングを同期させるため、
      | マグネットクラッチON/OFFをコントロールする。
  xcolc : Inport
  xacct1 : Inport  Port=2
  ne : Inport  Port=3
  xrload : Inport  Port=4
  w_tsmpl : Inport  Port=5
  rq_did_099b_b05_i : Inport  Port=6
  xdid_099b_b05_i : Inport  Port=7
  xenst : Inport  Port=8
  w_xsdpan : Inport  Port=9
  tqe_rsv_ac : Inport  Port=10
  Constant1 : lib2011b/Simulink Original/Sources/MC_Constant  Value=0  datatype=single  SampleTime=inf  FramePeriod=inf  OutMin=[]  OutMax=[]  OutDataTypeStr=single
  Constant12 : lib2011b/Simulink Original/Sources/MC_Constant  Value=false  datatype=Inherit: Inherit from 'Constant value'  SampleTime=inf  FramePeriod=inf  OutMin=[]  OutMax=[]  OutDataTypeStr=Inherit: Inherit from 'Constant value'
  Constant27 : lib2011b/Simulink Original/Sources/MC_Constant  Value=0  datatype=single  SampleTime=inf  FramePeriod=inf  OutMin=[]  OutMax=[]  OutDataTypeStr=single
  DownTimer_cnt15 : lib2011b/Mazda Library/Timer/MC_DownCountTimer
      settings: AttributesFormatString=DownCountTimer
  DownTimer_cnt16 : lib2011b/Mazda Library/Timer/MC_DownCountTimer
      settings: AttributesFormatString=DownCountTimer
  LogicalOperator1 : lib2011b/Simulink Original/Logic and Bit Operations/MC_LogicalOperator  SelectedOperator=NOT  Inputs=1  SampleTime=-1  AllPortsSameDT=off  OutDataTypeStr=boolean
  LogicalOperator2 : lib2011b/Simulink Original/Logic and Bit Operations/MC_LogicalOperator  SelectedOperator=OR  Inputs=2  SampleTime=-1  AllPortsSameDT=off  OutDataTypeStr=boolean
  LogicalOperator3 : lib2011b/Simulink Original/Logic and Bit Operations/MC_LogicalOperator  SelectedOperator=AND  Inputs=2  SampleTime=-1  AllPortsSameDT=off  OutDataTypeStr=boolean
  LogicalOperator4 : lib2011b/Simulink Original/Logic and Bit Operations/MC_LogicalOperator  SelectedOperator=NOT  Inputs=1  SampleTime=-1  AllPortsSameDT=off  OutDataTypeStr=boolean
  LogicalOperator42 : lib2011b/Simulink Original/Logic and Bit Operations/MC_LogicalOperator  SelectedOperator=NOT  Inputs=1  SampleTime=-1  AllPortsSameDT=off  OutDataTypeStr=boolean
  LogicalOperator5 : lib2011b/Simulink Original/Logic and Bit Operations/MC_LogicalOperator  SelectedOperator=OR  Inputs=2  SampleTime=-1  AllPortsSameDT=off  OutDataTypeStr=boolean
  MC_Constant : lib2011b/Simulink Original/Sources/MC_Constant  Value=KDP0532SP  datatype=Inherit: Inherit from 'Constant value'  SampleTime=inf  FramePeriod=inf  OutMin=[]  OutMax=[]  OutDataTypeStr=Inherit: Inherit from 'Constant value'
  MC_Constant1 : lib2011b/Simulink Original/Sources/MC_Constant  Value=0  datatype=uint8  SampleTime=inf  FramePeriod=inf  OutMin=[]  OutMax=[]  OutDataTypeStr=uint8
  MC_Constant2 : lib2011b/Simulink Original/Sources/MC_Constant  Value=KACC_FORCEDACON  datatype=Inherit: Inherit from 'Constant value'  SampleTime=inf  FramePeriod=inf  OutMin=[]  OutMax=[]  OutDataTypeStr=Inherit: Inherit from 'Constant value'
  MC_DataTypeConversion : lib2011b/Simulink Original/Signal Attributes/MC_DataTypeConversion  OutMin=[]  OutMax=[]  OutDataTypeStr=boolean  Signaltype=boolean  ConvertRealWorld=Real World Value (RWV)  RndMeth=Zero  SampleTime=-1
  MC_Edge1 : SUBSYSTEM_LIB_CNV/FallEdge
      settings: AttributesFormatString=FALL
  MC_Edge6 : SUBSYSTEM_LIB_CNV/RiseEdge
      settings: AttributesFormatString=RISE
  MC_LogicalOperator : lib2011b/Simulink Original/Logic and Bit Operations/MC_LogicalOperator  SelectedOperator=AND  Inputs=2  SampleTime=-1  AllPortsSameDT=off  OutDataTypeStr=boolean
  MC_LogicalOperator1 : lib2011b/Simulink Original/Logic and Bit Operations/MC_LogicalOperator  SelectedOperator=AND  Inputs=2  SampleTime=-1  AllPortsSameDT=off  OutDataTypeStr=boolean
  MC_LogicalOperator2 : lib2011b/Simulink Original/Logic and Bit Operations/MC_LogicalOperator  SelectedOperator=NOT  Inputs=2  SampleTime=-1  AllPortsSameDT=off  OutDataTypeStr=boolean
  MC_RelationalOperator : lib2011b/Simulink Original/Logic and Bit Operations/MC_RelationalOperator  Operator=>  SampleTime=-1  InputSameDT=on  OutDataTypeStr=boolean
  MC_Rename : lib2011b/Mazda Library/Other/MC_Rename
  MC_SID2F_B : lib2011b/Mazda Library/ServiceTool/MC_SID2F_B
      settings: AttributesFormatString=boolean
  MC_SetFlag : lib2011b/Mazda Library/Other/MC_SetFlag
      settings: AttributesFormatString=SetFlag
  MC_UnitDelay : lib2011b/Simulink Original/Discrete/MC_UnitDelay  InitialCondition=0  InputProcessing=Inherited  SampleTime=-1  StateName=delay_yclcn_b20m9500
      settings: StateMustResolveToSignalObject=off  StateStorageClass=ExportedGlobal
  MC_UnitDelay1 : lib2011b/Simulink Original/Discrete/MC_UnitDelay  InitialCondition=0  InputProcessing=Inherited  SampleTime=-1  StateName=delay_yclcn_b20m9501
      settings: StateMustResolveToSignalObject=off  StateStorageClass=ExportedGlobal
  RelationalOperator12 : lib2011b/Simulink Original/Logic and Bit Operations/MC_RelationalOperator  Operator=<=  SampleTime=-1  InputSameDT=on  OutDataTypeStr=boolean
  RelationalOperator13 : lib2011b/Simulink Original/Logic and Bit Operations/MC_RelationalOperator  Operator=<=  SampleTime=-1  InputSameDT=on  OutDataTypeStr=boolean
  set_init1 : Subsystem
  set_init2 : Subsystem
  xclcn : Outport
  clacdf : Outport  Port=2
  clacdl : Outport  Port=3
  xdid_099b_b05_r : Outport  Port=4
  xe_did_099b_b05 : Outport  Port=5
  xsp_did_099b_b05 : Outport  Port=6
  wires:
  set_init1/1(w_init) -> DownTimer_cnt15/4
  LogicalOperator2/1 -> DownTimer_cnt15/1
  LogicalOperator3/1 -> LogicalOperator2/1
  w_xsdpan/1 -> LogicalOperator2/2
  [xrload] -> set_init2/2(xrload)
  [ne] -> set_init2/1(ne)
  [xrload] -> set_init1/2(xrload)
  [ne] -> set_init1/1(ne)
  w_tsmpl/1 -> [w_tsmpl]  "w_tsmpl"
  ne/1 -> [ne]
  xrload/1 -> [xrload]
  xcolc/1 -> MC_LogicalOperator/1, MC_LogicalOperator2/1, [xcolc]
  Constant12/1 -> DownTimer_cnt16/1
  [w_tsmpl] -> DownTimer_cnt16/5
  [w_tsmpl] -> DownTimer_cnt15/5
  Constant27/1 -> RelationalOperator12/2
  DownTimer_cnt15/1 -> clacdf/1, RelationalOperator12/1  "clacdf"
  LogicalOperator1/1 -> LogicalOperator3/2
  Constant1/1 -> RelationalOperator13/2
  DownTimer_cnt16/1 -> RelationalOperator13/1, clacdl/1  "clacdl"
  LogicalOperator42/1 -> DownTimer_cnt15/3
  xacct1/1 -> LogicalOperator3/1
  set_init2/1(w_init) -> DownTimer_cnt16/4
  MC_SID2F_B/2 -> xdid_099b_b05_r/1  "xdid_099b_b05_r"
  MC_SID2F_B/1 -> xclcn/1, MC_UnitDelay/1  "xclcn"
  rq_did_099b_b05_i/1 -> MC_SID2F_B/1
  xdid_099b_b05_i/1 -> MC_SID2F_B/3
  xenst/1 -> MC_Rename/1
  MC_Rename/1 -> xe_did_099b_b05/1  "xe_did_099b_b05"
  MC_Constant/1 -> MC_RelationalOperator/1
  MC_Constant1/1 -> MC_RelationalOperator/2
  MC_RelationalOperator/1 -> xsp_did_099b_b05/1  "xsp_did_099b_b05"
  MC_LogicalOperator1/1 -> MC_SetFlag/1
  MC_LogicalOperator/1 -> MC_SetFlag/2
  MC_LogicalOperator2/1 -> MC_LogicalOperator1/2
  [xcolc] -> DownTimer_cnt16/3
  RelationalOperator12/1 -> MC_LogicalOperator1/1
  RelationalOperator13/1 -> MC_LogicalOperator/2
  [xcolc] -> LogicalOperator42/1
  [xcolc] -> LogicalOperator1/1
  MC_Edge1/1 -> DownTimer_cnt15/2, set_init1/Enable
  MC_Edge6/1 -> DownTimer_cnt16/2, set_init2/Enable
  [xcolc] -> MC_Edge1/1
  [xcolc] -> MC_Edge6/1
  MC_UnitDelay/1 -> [w_xclcn_lst]
  [w_xclcn_lst] -> MC_Edge6/2
  [w_xclcn_lst] -> LogicalOperator4/1
  LogicalOperator4/1 -> MC_Edge1/2
  MC_Constant2/1 -> MC_DataTypeConversion/1
  MC_SetFlag/1 -> LogicalOperator5/2
  LogicalOperator5/1 -> MC_SID2F_B/2
  MC_DataTypeConversion/1 -> LogicalOperator5/1
  tqe_rsv_ac/1 -> MC_UnitDelay1/1
  [tqe_rsv_ac] -> set_init1/3(tqe_rsv_ac)
  [tqe_rsv_ac] -> set_init2/3(tqe_rsv_ac)
  MC_UnitDelay1/1 -> [tqe_rsv_ac]
